simulink model "InertiaTensorCoordSysCalculator"  (R2021b)
settings: Solver=VariableStepAuto  StartTime=0.0  StopTime=10.0  RelTol=1e-3
settings Model: Creator=Ian Lee  LastModifiedBy=Ian Lee

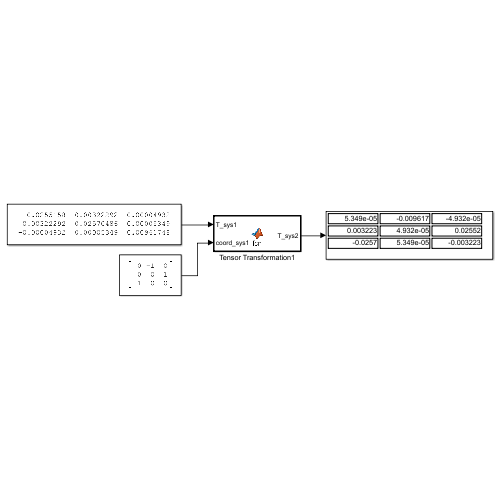
[thumbnail: Simulink's stored preview of the top-level diagram]
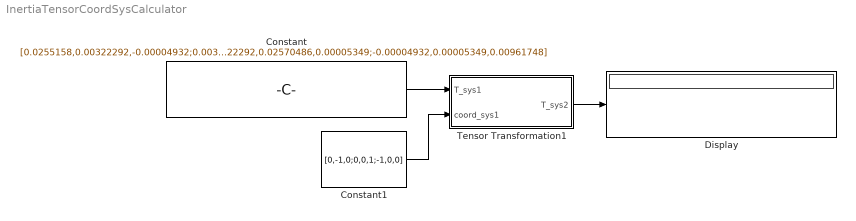
== system InertiaTensorCoordSysCalculator ==
  Constant : Constant  Value=[0.0255158,0.00322292,-0.00004932;0.00322292,0.02570486,0.00005349;-0.00004932,0.00005349,0.00961748]
  Constant1 : Constant  Value=[0,-1,0;0,0,1;-1,0,0]
  Display : Display
  Tensor Transformation1 : MATLAB Function  TreatAsAtomicUnit=on
  wires:
  Constant1/1 -> Tensor Transformation1/2(coord_sys1)
  Tensor Transformation1/1(T_sys2) -> Display/1
  Constant/1 -> Tensor Transformation1/1(T_sys1)

== matlab function InertiaTensorCoordSysCalculator/Tensor Transformation1 ==
  data: T_sys1 input; T_sys2 output; coord_sys1 input
% transform tensor from standard cartesian to another given rotated cartesian system unit
% vectors
function T_sys2 = fcn(T_sys1,coord_sys1)

% normalize coordinate systems
coord_sys1 = coord_sys1 / norm(coord_sys1);

c2 = [1,0,0;0,1,0;0,0,1];
c1 = coord_sys1;

trans_mat = [
dot(c2(1,:),c1(1,:)), dot(c2(1,:),c1(2,:)), dot(c2(1,:),c1(3,:));
dot(c2(2,:),c1(1,:)), dot(c2(2,:),c1(2,:)), dot(c2(2,:),c1(3,:));
dot(c2(3,:),c1(1,:)), dot(c2(3,:),c1(2,:)), dot(c2(3,:),c1(3,:));
];

T_sys2 = trans_mat * T_sys1;
T_sys2 = T_sys2 * trans_mat;
